simulink model "model"  (R2020b)
settings: Solver=VariableStepAuto  StartTime=0.0  StopTime=10.0  RelTol=1e-3
settings Model: Creator=Lenovo  LastModifiedBy=Lenovo

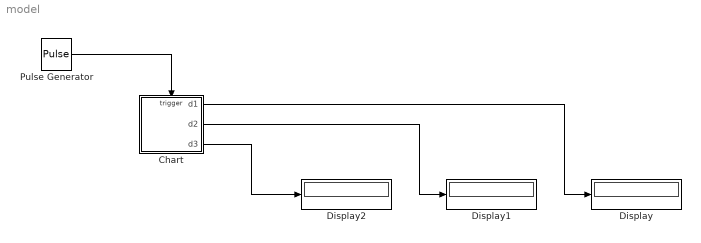
== system model ==
  Chart : Stateflow chart  TreatAsAtomicUnit=on
  Display : Display
  Display1 : Display
  Display2 : Display
  Pulse Generator : DiscretePulseGenerator  PulseType=Time based  Period=10  PulseWidth=5
  wires:
  Pulse Generator/1 -> Chart/Trigger
  Chart/3(d3) -> Display2/1
  Chart/2(d2) -> Display1/1
  Chart/1(d1) -> Display/1

== stateflow chart model/Chart ==
  data: d1 output; d2 output; d3 output
  events: Input_pulse input FUNCTION_CALL_EVENT
